simulink model "Host_handson"  (R2015b)
settings: Solver=FixedStepAuto  StartTime=0.0  StopTime=inf  RelTol=1e-3
libraries: c2000scilib x3, demo_controls x1
settings Model: Creator=aancelle  LastModifiedBy=ata.otaran
settings DataIOCC: SaveFormat=Array  SignalLoggingSaveFormat=ModelDataLogs
settings OptimizationCC: BlockReduction=off  OptimizeModelRefInitCode=on  LifeSpan=1
settings DebuggingCC: UnderspecifiedInitializationDetection=Classic  MergeDetectMultiDrivingBlocksExec=none  SolverPrmCheckMsg=warning
settings HardwareCC: ProdBitPerPointer=32  ProdLargestAtomicFloat=None  ProdIntDivRoundTo=Undefined  ProdEndianess=Unspecified  ProdWordSize=32  ProdHWDeviceType=32-bit Generic
settings RTWCC: SystemTargetFile=ert.tlc  TemplateMakefile=ert_default_tmf  Description=Real-Time Workshop Embedded Coder  GenerateReport=on  IncludeHyperlinkInReport=on  LaunchReport=on  GenerateTraceInfo=on  GenerateTraceReport=on  GenerateTraceReportSl=on  GenerateTraceReportSf=on  GenerateTraceReportEml=on
settings CodeAppCC: IgnoreCustomStorageClasses=off  InternalIdentifier=Classic
settings ERTTargetCC: GenerateSampleERTMain=on  ERTCustomFileTemplate=example_file_process.tlc
settings ConfigComp: CovModelRefEnable=Off

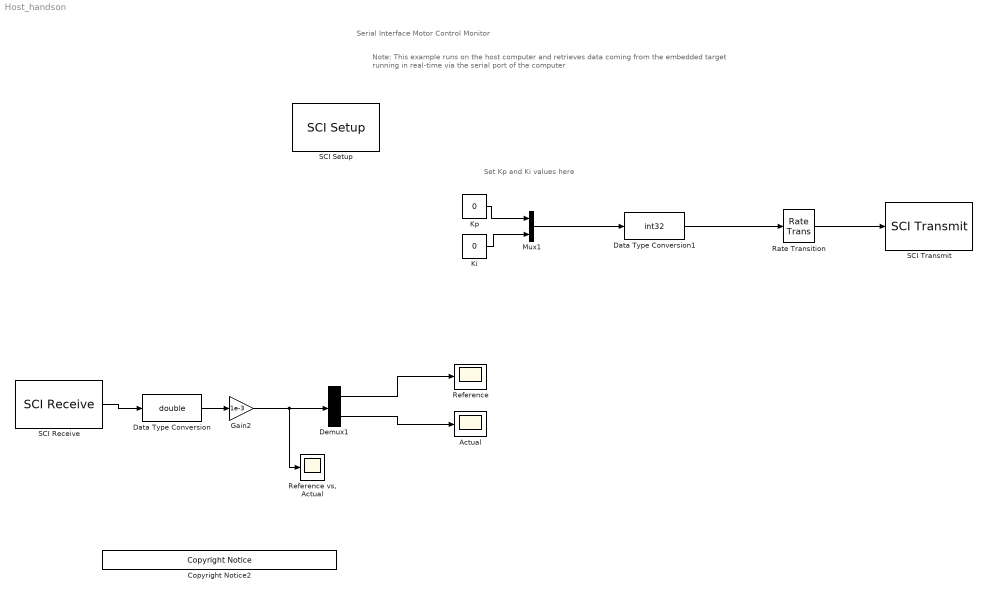
== system Host_handson ==
  note: Set Kp and Ki values here
  note: Note: This example runs on the host computer and retrieves data
      | coming from the embedded target running in real-time via the serial port of the computer
  note: Serial Interface Motor Control Monitor
  Actual : Scope
  Copyright Notice2 : demo_controls/Copyright Notice  year=2014  prod=tic2000
  Data Type Conversion : DataTypeConversion  OutDataTypeStr=double  ConvertRealWorld=Stored Integer (SI)
  Data Type Conversion1 : DataTypeConversion  OutDataTypeStr=int32  ConvertRealWorld=Stored Integer (SI)
  Demux1 : Demux  Outputs=2
  Gain2 : Gain  Gain=1e-3
  Ki : Constant  Value=0
  Kp : Constant  Value=0
  Mux1 : Mux  Inputs=2
  Rate Transition : RateTransition  OutPortSampleTime=0.05
  Reference : Scope
  "Reference vs, Actual" : Scope
  SCI Receive : c2000scilib/SCI Receive  module=COM 2  dataHead='S'  dataTail='E'  dataType=int32  dataDim=2  initValue=0  errOption=Output the last received value  errValue=0  sampleTime=0.01  outputStatus=off
  SCI Setup : c2000scilib/SCI Setup  Priority=-99  commModeA=raw data  baudRateA=115200  charLenA=8  stopBitA=1  parityA=none  timeoutA=1.0  commModeB=raw data  baudRateB=115200  charLenB=8  stopBitB=1  parityB=none  timeoutB=1.0  commModeC=raw data  baudRateC=115200  charLenC=8  stopBitC=1  parityC=none  timeoutC=1.0  commModeD=raw data  baudRateD=115200  charLenD=8  stopBitD=1  parityD=none  timeoutD=1.0
  SCI Transmit : c2000scilib/SCI Transmit  module=COM 2  header='S'  tail='E'
  wires:
  SCI Receive/1 -> Data Type Conversion/1
  Data Type Conversion/1 -> Gain2/1
  Mux1/1 -> Data Type Conversion1/1
  Ki/1 -> Mux1/2
  Kp/1 -> Mux1/1
  Gain2/1 -> "Reference vs, Actual"/1, Demux1/1
  Data Type Conversion1/1 -> Rate Transition/1
  Rate Transition/1 -> SCI Transmit/1
  Demux1/1 -> Reference/1
  Demux1/2 -> Actual/1
